simulink model "task_2"  (R2024a)
settings: Solver=VariableStepAuto  StartTime=0.0  StopTime=10.0  RelTol=1e-3
settings Model: Creator=alexe  LastModifiedBy=alexe

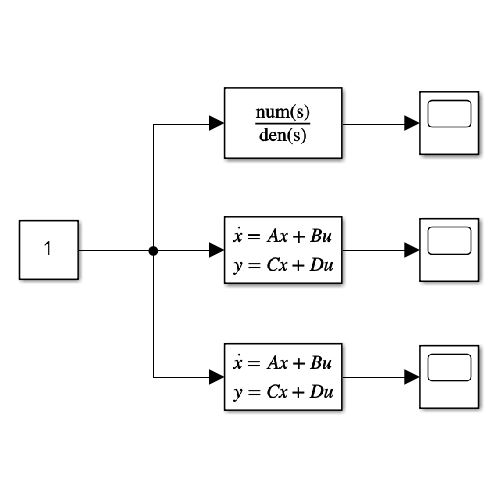
[thumbnail: Simulink's stored preview of the top-level diagram]
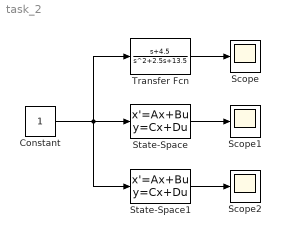
== system task_2 ==
  Constant : Constant
  Scope : Scope
  Scope1 : Scope
  Scope2 : Scope
  State-Space : StateSpace  A=[0 1; -13.5 -2.5]  B=[0;1]  C=[4.5 1]  D=0  InitialCondition=0
  State-Space1 : StateSpace  A=[0 -13.5; 1 -2.5]  B=[4.5;1]  C=[0 1]  D=0  InitialCondition=0
  Transfer Fcn : TransferFcn  Numerator=[1 4.5]  Denominator=[1 2.5 13.5]
  wires:
  Constant/1 -> State-Space1/1, State-Space/1, Transfer Fcn/1
  Transfer Fcn/1 -> Scope/1
  State-Space/1 -> Scope1/1
  State-Space1/1 -> Scope2/1
